simulink model "steadystatesimulink"  (R2025b)
settings: Solver=VariableStepAuto  StartTime=0.0  StopTime=0.5  RelTol=1e-3
settings Model: Creator=mulua  LastModifiedBy=mulua

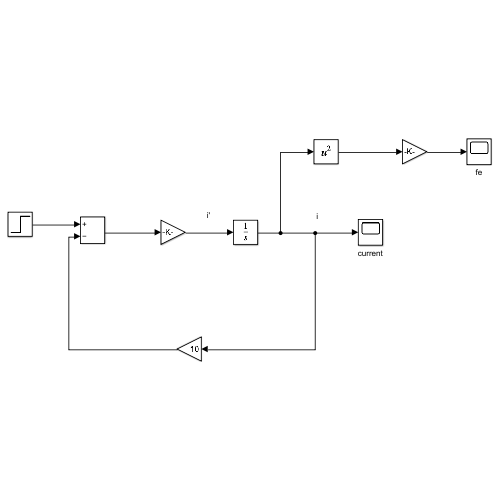
[thumbnail: Simulink's stored preview of the top-level diagram]
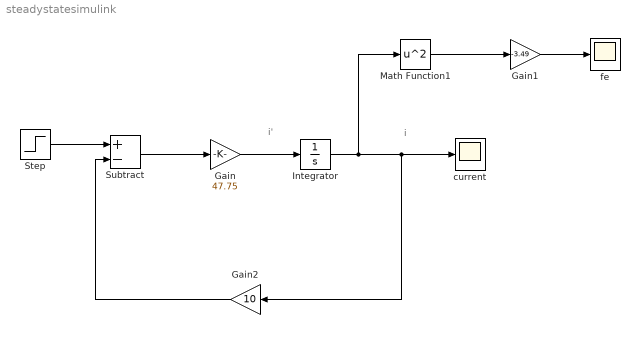
== system steadystatesimulink ==
  note: i
  note: i'
  Gain : Gain  Gain=47.75
  Gain1 : Gain  Gain=-3.49
  Gain2 : Gain  Gain=10
  Integrator : Integrator
  Math Function1 : Math  Operator=square
  Step : Step  Time=0  After=5  SampleTime=0
  Subtract : Sum  Inputs=+-
  current : Scope
      settings: ActiveDisplayYMinimum=-0.062495028331112361  ActiveDisplayYMaximum=0.56245525498001137
  fe : Scope
      settings: ActiveDisplayYMinimum=-0.981406346091251  ActiveDisplayYMaximum=0.10904514956569453  DataLoggingVariableName=ScopeData2
  wires:
  Step/1 -> Subtract/1
  Subtract/1 -> Gain/1
  Gain/1 -> Integrator/1
  Integrator/1 -> Math Function1/1, Gain2/1, current/1
  Math Function1/1 -> Gain1/1
  Gain2/1 -> Subtract/2
  Gain1/1 -> fe/1
